simulink model "srm"  (R2013b)
settings: Solver=ode45  StartTime=0.0  StopTime=3  MaxStep=1e-4  RelTol=1e-3
InitFcn:
  | iref=30;
settings Model: Creator=Think79  LastModifiedBy=Think79
settings ConfigurationSet: Description=SimMechanics 2G

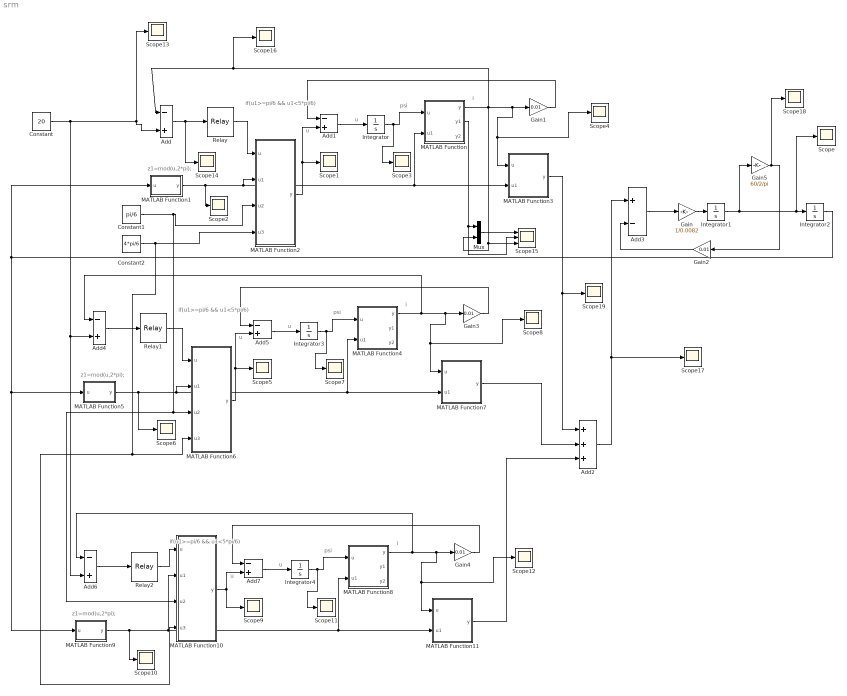
== system srm ==
  note: u
  note: z1=mod(u,2*pi);
  note: if(u1>=pi/6 && u1<5*pi/6)
  note: i
  note: psi
  note: u
  note: u
  note: z1=mod(u,2*pi);
  note: if(u1>=pi/6 && u1<5*pi/6)
  note: i
  note: psi
  note: u
  note: u
  note: z1=mod(u,2*pi);
  note: if(u1>=pi/6 && u1<5*pi/6)
  note: i
  note: psi
  note: u
  Add{,1,4..7} (6 alike) : Sum  Inputs=-+
  Add2 : Sum  Inputs=+++
  Add3 : Sum  Inputs=+-
  Constant : Constant  Value=20
  Constant1 : Constant  Value=pi/6
  Constant2 : Constant  Value=4*pi/6
  Gain : Gain  Gain=1/0.0082
  Gain{1..4} (4 alike) : Gain  Gain=0.01
  Gain5 : Gain  Gain=60/2/pi
  Integrator : Integrator  LimitOutput=on  LowerSaturationLimit=0
  Integrator1 : Integrator
  Integrator2 : Integrator  InitialCondition=pi/6
  Integrator3 : Integrator  LimitOutput=on  LowerSaturationLimit=0
  Integrator4 : Integrator  LimitOutput=on  LowerSaturationLimit=0
  MATLAB Function : MATLAB Function  TreatAsAtomicUnit=on
  MATLAB Function1 : MATLAB Function  TreatAsAtomicUnit=on
  MATLAB Function10 : MATLAB Function  TreatAsAtomicUnit=on
  MATLAB Function11 : MATLAB Function  TreatAsAtomicUnit=on
  MATLAB Function2 : MATLAB Function  TreatAsAtomicUnit=on
  MATLAB Function3 : MATLAB Function  TreatAsAtomicUnit=on
  MATLAB Function4 : MATLAB Function  TreatAsAtomicUnit=on
  MATLAB Function5 : MATLAB Function  TreatAsAtomicUnit=on
  MATLAB Function6 : MATLAB Function  TreatAsAtomicUnit=on
  MATLAB Function7 : MATLAB Function  TreatAsAtomicUnit=on
  MATLAB Function8 : MATLAB Function  TreatAsAtomicUnit=on
  MATLAB Function9 : MATLAB Function  TreatAsAtomicUnit=on
  Mux : Mux  Inputs=2
  Relay : Relay  OnSwitchValue=1  OffSwitchValue=-1  OnOutputValue=240  OffOutputValue=-240
  Relay1 : Relay  OnSwitchValue=1  OffSwitchValue=-1  OnOutputValue=240  OffOutputValue=-240
  Relay2 : Relay  OnSwitchValue=1  OffSwitchValue=-1  OnOutputValue=240  OffOutputValue=-240
  Scope{,1..14,16..19} (19 alike) : Scope
      Scope10 settings: SaveName=ScopeData9
      Scope11 settings: SaveName=ScopeData10
      Scope12 settings: SaveName=ScopeData11
      Scope13 settings: SaveName=ScopeData13
      Scope14 settings: SaveName=ScopeData14
      Scope16 settings: TimeRange=0.002748230455929455  YMin=0  YMax=35  SaveName=ScopeData16
      Scope17 settings: SaveName=ScopeData17
      Scope18 settings: YMin=-3.36042e-25  YMax=2.1e-09  SaveName=ScopeData18
      Scope19 settings: SaveName=ScopeData19
      Scope2 settings: SaveName=ScopeData2
      Scope3 settings: SaveName=ScopeData3
      Scope4 settings: SaveName=ScopeData4
      Scope5 settings: SaveName=ScopeData5
      Scope6 settings: SaveName=ScopeData6
      Scope7 settings: SaveName=ScopeData7
      Scope8 settings: SaveName=ScopeData8
      Scope9 settings: SaveName=ScopeData12
  Scope15 : Scope  NumInputPorts=3
      settings: YMin=-5~-5~-5  YMax=5~5~5  SaveName=ScopeData15
  wires:
  Add/1 -> Scope14/1, Relay/1
  Integrator1/1 -> Gain5/1, Integrator2/1, Scope/1
  MATLAB Function2/1(y) -> Add1/2, Scope1/1
  Add1/1 -> Integrator/1
  MATLAB Function1/1(y) -> Scope2/1, MATLAB Function3/2(u1), MATLAB Function/2(u1), MATLAB Function2/2(u1)
  Relay/1 -> MATLAB Function2/1(u)
  Integrator/1 -> Scope3/1, MATLAB Function/1(u)
  MATLAB Function/1(y) -> Scope15/3, Mux/2, Scope16/1, Add/1, Scope4/1, MATLAB Function3/1(u), Gain1/1
  MATLAB Function3/1(y) -> Scope19/1, Add2/1
  Add2/1 -> Scope17/1, Add3/1
  Add3/1 -> Gain/1
  Gain1/1 -> Add1/1
  Gain2/1 -> Add3/2
  Integrator2/1 -> MATLAB Function1/1(u), MATLAB Function9/1(u), MATLAB Function5/1(u)
  Gain/1 -> Integrator1/1
  Add4/1 -> Relay1/1
  MATLAB Function6/1(y) -> Add5/2, Scope5/1
  Add5/1 -> Integrator3/1
  MATLAB Function5/1(y) -> Scope6/1, MATLAB Function6/2(u1), MATLAB Function7/2(u1), MATLAB Function4/2(u1)
  Relay1/1 -> MATLAB Function6/1(u)
  Integrator3/1 -> Scope7/1, MATLAB Function4/1(u)
  MATLAB Function4/1(y) -> Add4/1, Scope8/1, MATLAB Function7/1(u), Gain3/1
  Gain3/1 -> Add5/1
  MATLAB Function7/1(y) -> Add2/2
  Constant/1 -> Add6/2, Add4/2, Add/2, Scope13/1
  Add6/1 -> Relay2/1
  MATLAB Function10/1(y) -> Scope9/1, Add7/2
  Add7/1 -> Integrator4/1
  MATLAB Function9/1(y) -> Scope10/1, MATLAB Function10/2(u1), MATLAB Function11/2(u1), MATLAB Function8/2(u1)
  Relay2/1 -> MATLAB Function10/1(u)
  Integrator4/1 -> Scope11/1, MATLAB Function8/1(u)
  MATLAB Function8/1(y) -> Add6/1, Scope12/1, MATLAB Function11/1(u), Gain4/1
  Gain4/1 -> Add7/1
  MATLAB Function11/1(y) -> Add2/3
  MATLAB Function/2(y1) -> Scope15/2, Mux/1
  Gain5/1 -> Scope18/1, Gain2/1
  Constant1/1 -> MATLAB Function10/3(u2), MATLAB Function6/3(u2), MATLAB Function2/3(u2)
  Constant2/1 -> MATLAB Function6/4(u3), MATLAB Function10/4(u3), MATLAB Function2/4(u3)
  Mux/1 -> Scope15/1

== matlab function srm/MATLAB Function1 ==
  data: u input; y output
function y  = fcn(u)
z1=0;
z1=u*8;
z1=mod(u,2*pi);
%不同的相z1要减去不同的值
y=z1;

end

== matlab function srm/MATLAB Function ==
  data: u input; y output; u1 input; y1 output; y2 output
function [y,y1,y2] = fcn(u,   u1)
y=0;
y1=0;
y2=0;
if(u1>=pi/6 && u1<5*pi/6)
    L=(u1-pi/6)*(0.007*6/4/pi)+0.005;
elseif(u1>=7*pi/6 && u1<11*pi/6)
    L=-(u1-11*pi/6)*(0.007*6/4/pi)+0.005;
elseif(u1>=5*pi/6 && u1<7*pi/6)
    L=0.012;
else
    L=0.005;
end
y=u/L;
y1=L;    

end

== matlab function srm/MATLAB Function2 ==
  data: u input; y output; u1 input; u2 input; u3 input
function y  = fcn(u,u1,u2,u3)
if(u1>=u2 && u1<u3)
    y=u;
else
    y=-abs(u);
end


end

== matlab function srm/MATLAB Function3 ==
  data: u input; y output; u1 input
function y  = fcn(u,   u1)
if(u1>=pi/6 && u1<5*pi/6)
    a1=1;
elseif(u1>=7*pi/6 && u1<11*pi/6)
        a1=-1;

else
    a1=0;
end
y=a1*(8/300)*u*u;
end

== matlab function srm/MATLAB Function4 ==
  data: u input; y output; u1 input; y1 output; y2 output
function [y,y1,y2] = fcn(u,   u1)
y=0;
y1=0;
y2=0;
if(u1>=pi/6 && u1<5*pi/6)
    L=(u1-pi/6)*(0.007*6/4/pi)+0.005;
elseif(u1>=7*pi/6 && u1<11*pi/6)
    L=-(u1-11*pi/6)*(0.007*6/4/pi)+0.005;
elseif(u1>=5*pi/6 && u1<7*pi/6)
    L=0.012;
else
    L=0.005;
end
y=u/L;
    

end

== matlab function srm/MATLAB Function5 ==
  data: u input; y output
function y  = fcn(u)
z1=0;
z1=u*8;
z1=mod(u,2*pi);
%不同的相z1要减去不同的值
z1=z1-4*pi/6;
if(z1<0)
    z1=z1+2*pi;
else
end
y=z1;

end

== matlab function srm/MATLAB Function6 ==
  data: u input; y output; u1 input; u2 input; u3 input
function y  = fcn(u,u1,u2,u3)
if(u1>=u2 && u1<u3)
    y=u;
else
    y=-abs(u);
end


end

== matlab function srm/MATLAB Function7 ==
  data: u input; y output; u1 input
function y  = fcn(u,   u1)
if(u1>=pi/6 && u1<5*pi/6)
    a1=1;
elseif(u1>=7*pi/6 && u1<11*pi/6)
        a1=-1;

else
    a1=0;
end
y=a1*(8/300)*u*u;
end

== matlab function srm/MATLAB Function10 ==
  data: u input; y output; u1 input; u2 input; u3 input
function y  = fcn(u,u1,u2,u3)
if(u1>=u2 && u1<u3)
    y=u;
else
    y=-abs(u);
end


end

== matlab function srm/MATLAB Function11 ==
  data: u input; y output; u1 input
function y  = fcn(u,   u1)
if(u1>=pi/6 && u1<5*pi/6)
    a1=1;
elseif(u1>=7*pi/6 && u1<11*pi/6)
        a1=-1;

else
    a1=0;
end
y=a1*(8/300)*u*u;
end

== matlab function srm/MATLAB Function8 ==
  data: u input; y output; u1 input; y1 output; y2 output
function [y,y1,y2] = fcn(u,   u1)
y=0;
y1=0;
y2=0;
if(u1>=pi/6 && u1<5*pi/6)
    L=(u1-pi/6)*(0.007*6/4/pi)+0.005;
elseif(u1>=7*pi/6 && u1<11*pi/6)
    L=-(u1-11*pi/6)*(0.007*6/4/pi)+0.005;
elseif(u1>=5*pi/6 && u1<7*pi/6)
    L=0.012;
else
    L=0.005;
end
y=u/L;
    

end

== matlab function srm/MATLAB Function9 ==
  data: u input; y output
function y  = fcn(u)
z1=0;
z1=u*8;
z1=mod(u,2*pi);
%不同的相z1要减去不同的值
z1=z1-8*pi/6;
if(z1<0)
    z1=z1+2*pi;
else
end
y=z1;

end
